simulink model "problema1a"  (R2019a)
settings: Solver=FixedStepDiscrete  StartTime=0.0  StopTime=10.0  FixedStep=1  RelTol=1e-3
libraries: simulink x1
settings Model: Creator=prestamour  LastModifiedBy=prestamour

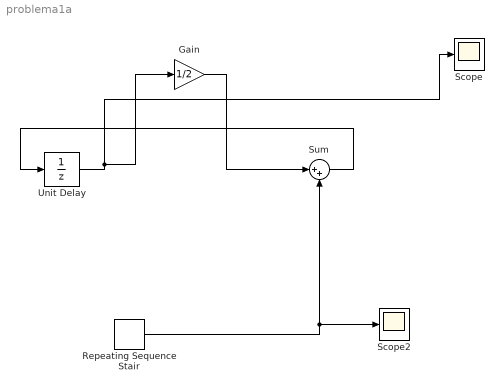
== system problema1a ==
  Gain : Gain  Gain=1/2
  Repeating Sequence Stair : simulink/Sources/Repeating Sequence Stair  OutValues="[0 1 1 1 1 0 0 0 0 0 0 0 0 0 0 0 0 0 0  ].'"  tsamp=-1  OutMin=[]  OutMax=[]  OutDataTypeStr=double  OutputDataTypeScalingMode=double  OutDataType=fixdt(0,8)  ConRadixGroup=Best Precision: Vector-wise  OutScaling=2^-12
  Scope : Scope
  Scope2 : Scope
  Sum : Sum  Inputs=|++
  Unit Delay : UnitDelay  InitialCondition=1  SampleTime=-1  HasFrameUpgradeWarning=on
  wires:
  Unit Delay/1 -> Scope/1, Gain/1
  Gain/1 -> Sum/1
  Repeating Sequence Stair/1 -> Scope2/1, Sum/2
  Sum/1 -> Unit Delay/1
